simulink model "Battery_Pack_Subsystem"  (R2015a)
settings: Solver=ode45  StartTime=0.0  StopTime=300  RelTol=1e-3
libraries: fl_lib x316, nesl_utility x2
(part 1 of 2)
settings Model: Creator=satya  LastModifiedBy=satya

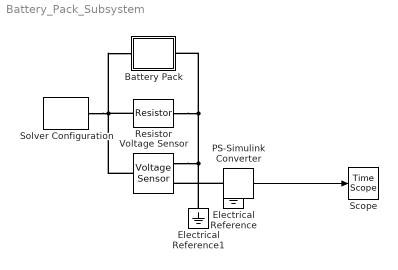
== system Battery_Pack_Subsystem ==
  Battery Pack : Subsystem
  Electrical Reference : fl_lib/Electrical/Electrical Elements/Electrical Reference
  Electrical Reference1 : fl_lib/Electrical/Electrical Elements/Electrical Reference
  PS-Simulink Converter : nesl_utility/PS-Simulink Converter  PhysicalDomain=network_engine_domain  SubClassName=ps_output  LeftPortType=input  RightPortType=output  PseudoPeriodic=off  Frequencies=[]  Unit=1  AffineConversion=off
  Resistor : fl_lib/Electrical/Electrical Elements/Resistor  R=1000 Ohm  i_specify=off  i_priority=High  i=0 A  v_specify=off  v_priority=High  v=0 V
  Scope : TimeScope
  Solver Configuration : nesl_utility/Solver Configuration  PhysicalDomain=network_engine_domain  SubClassName=solver  LeftPortType=input  RightPortType=generic  Accelerate=off  Tones=[]  Harmonics=[]  SimulateNoise=off  Profile=off  UseLocalSampling=off  EnableSwitchedLinearOptims=on  FrequencyDomain=off  UseCCode=off  RelTol=0.001  AbsTol=1e-06  MinStep=1e-09  ToWorkspace=off  RevertToSquareIcSolve=off  NumHomotopyIterations=100  DoDC=off  ResidualTolerance=1e-09  UseLocalSolver=off  LocalSolverChoice=NE_BACKWARD_EULER_ADVANCER  LocalSolverSampleTime=0.001  DoFixedCost=off  MaxNonlinIter=3  MaxModeIter=2  LinearAlgebra=Sparse  DelaysMemoryBudget=1024  AutomaticFiltering=on  FilteringTimeConstant=0.001
  Voltage Sensor : fl_lib/Electrical/Electrical Sensors/Voltage Sensor
  wires:
  PS-Simulink Converter/1 -> Scope/1
  connections:
  Voltage Sensor/RConn2 -- Battery Pack/RConn1 -- Resistor/RConn1 -- Electrical Reference1/LConn1
  Voltage Sensor/LConn1 -- Battery Pack/LConn1 -- Resistor/LConn1 -- Solver Configuration/RConn1
  PS-Simulink Converter/LConn1 -- Voltage Sensor/RConn1

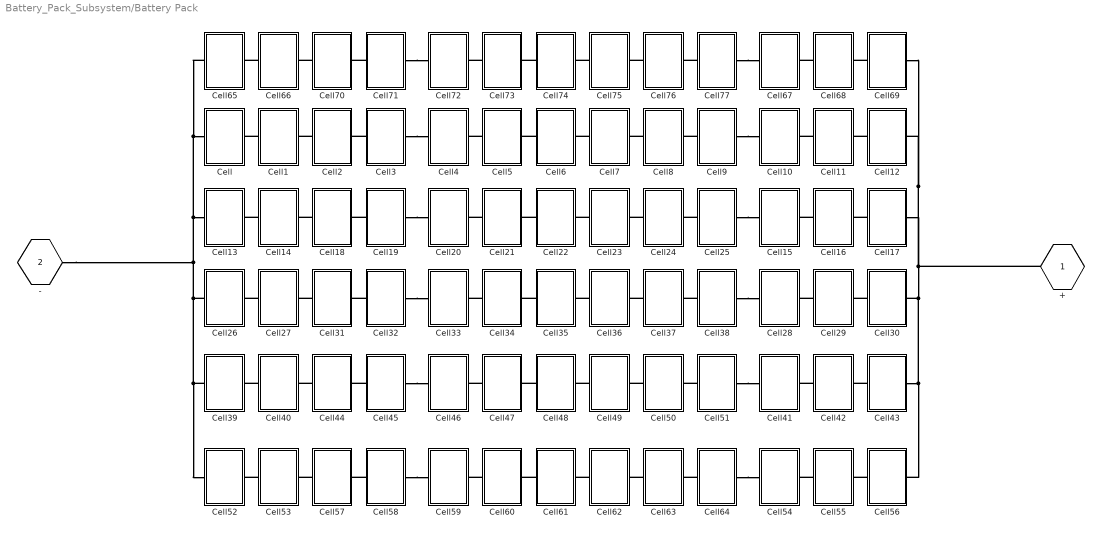
== system Battery_Pack_Subsystem/Battery Pack ==
  Cell : Subsystem
  Cell1 : Subsystem
  Cell10 : Subsystem
  Cell11 : Subsystem
  Cell12 : Subsystem
  Cell13 : Subsystem
  Cell14 : Subsystem
  Cell15 : Subsystem
  Cell16 : Subsystem
  Cell17 : Subsystem
  Cell18 : Subsystem
  Cell19 : Subsystem
  Cell2 : Subsystem
  Cell20 : Subsystem
  Cell21 : Subsystem
  Cell22 : Subsystem
  Cell23 : Subsystem
  Cell24 : Subsystem
  Cell25 : Subsystem
  Cell26 : Subsystem
  Cell27 : Subsystem
  Cell28 : Subsystem
  Cell29 : Subsystem
  Cell3 : Subsystem
  Cell30 : Subsystem
  Cell31 : Subsystem
  Cell32 : Subsystem
  Cell33 : Subsystem
  Cell34 : Subsystem
  Cell35 : Subsystem
  Cell36 : Subsystem
  Cell37 : Subsystem
  Cell38 : Subsystem
  Cell39 : Subsystem
  Cell4 : Subsystem
  Cell40 : Subsystem
  Cell41 : Subsystem
  Cell42 : Subsystem
  Cell43 : Subsystem
  Cell44 : Subsystem
  Cell45 : Subsystem
  Cell46 : Subsystem
  Cell47 : Subsystem
  Cell48 : Subsystem
  Cell49 : Subsystem
  Cell5 : Subsystem
  Cell50 : Subsystem
  Cell51 : Subsystem
  Cell52 : Subsystem
  Cell53 : Subsystem
  Cell54 : Subsystem
  Cell55 : Subsystem
  Cell56 : Subsystem
  Cell57 : Subsystem
  Cell58 : Subsystem
  Cell59 : Subsystem
  Cell6 : Subsystem
  Cell60 : Subsystem
  Cell61 : Subsystem
  Cell62 : Subsystem
  Cell63 : Subsystem
  Cell64 : Subsystem
  Cell65 : Subsystem
  Cell66 : Subsystem
  Cell67 : Subsystem
  Cell68 : Subsystem
  Cell69 : Subsystem
  Cell7 : Subsystem
  Cell70 : Subsystem
  Cell71 : Subsystem
  Cell72 : Subsystem
  Cell73 : Subsystem
  Cell74 : Subsystem
  Cell75 : Subsystem
  Cell76 : Subsystem
  Cell77 : Subsystem
  Cell8 : Subsystem
  Cell9 : Subsystem
  + : PMIOPort  Port=1  Side=Left
  - : PMIOPort  Port=2  Side=Right
  connections:
  Cell60/LConn1 -- Cell59/RConn1
  Cell62/LConn1 -- Cell61/RConn1
  Cell57/LConn1 -- Cell53/RConn1
  Cell64/RConn1 -- Cell54/LConn1
  Cell58/RConn1 -- Cell59/LConn1
  Cell64/LConn1 -- Cell63/RConn1
  Cell55/LConn1 -- Cell54/RConn1
  Cell63/LConn1 -- Cell62/RConn1
  Cell53/LConn1 -- Cell52/RConn1
  Cell58/LConn1 -- Cell57/RConn1
  Cell56/LConn1 -- Cell55/RConn1
  Cell61/LConn1 -- Cell60/RConn1
  Cell29/LConn1 -- Cell28/RConn1
  Cell31/LConn1 -- Cell27/RConn1
  Cell34/LConn1 -- Cell33/RConn1
  Cell35/LConn1 -- Cell34/RConn1
  Cell36/LConn1 -- Cell35/RConn1
  Cell32/LConn1 -- Cell31/RConn1
  Cell37/LConn1 -- Cell36/RConn1
  Cell38/RConn1 -- Cell28/LConn1
  Cell38/LConn1 -- Cell37/RConn1
  Cell51/LConn1 -- Cell50/RConn1
  Cell50/LConn1 -- Cell49/RConn1
  Cell51/RConn1 -- Cell41/LConn1
  Cell27/LConn1 -- Cell26/RConn1
  Cell40/LConn1 -- Cell39/RConn1
  Cell43/LConn1 -- Cell42/RConn1
  Cell45/RConn1 -- Cell46/LConn1
  Cell32/RConn1 -- Cell33/LConn1
  Cell30/LConn1 -- Cell29/RConn1
  Cell5/LConn1 -- Cell4/RConn1
  Cell47/LConn1 -- Cell46/RConn1
  Cell44/LConn1 -- Cell40/RConn1
  Cell48/LConn1 -- Cell47/RConn1
  Cell42/LConn1 -- Cell41/RConn1
  Cell49/LConn1 -- Cell48/RConn1
  Cell45/LConn1 -- Cell44/RConn1
  Cell2/LConn1 -- Cell1/RConn1
  Cell3/LConn1 -- Cell2/RConn1
  Cell77/LConn1 -- Cell76/RConn1
  Cell77/RConn1 -- Cell67/LConn1
  Cell71/LConn1 -- Cell70/RConn1
  Cell66/LConn1 -- Cell65/RConn1
  Cell76/LConn1 -- Cell75/RConn1
  Cell69/LConn1 -- Cell68/RConn1
  Cell71/RConn1 -- Cell72/LConn1
  Cell74/LConn1 -- Cell73/RConn1
  Cell73/LConn1 -- Cell72/RConn1
  Cell68/LConn1 -- Cell67/RConn1
  Cell70/LConn1 -- Cell66/RConn1
  Cell75/LConn1 -- Cell74/RConn1
  Cell6/LConn1 -- Cell5/RConn1
  Cell11/LConn1 -- Cell10/RConn1
  Cell7/LConn1 -- Cell6/RConn1
  Cell8/LConn1 -- Cell7/RConn1
  Cell9/RConn1 -- Cell10/LConn1
  Cell9/LConn1 -- Cell8/RConn1
  Cell43/RConn1 -- Cell56/RConn1 -- +/RConn1 -- Cell17/RConn1 -- Cell69/RConn1 -- Cell12/RConn1 -- Cell30/RConn1
  Cell3/RConn1 -- Cell4/LConn1
  Cell12/LConn1 -- Cell11/RConn1
  Cell25/RConn1 -- Cell15/LConn1
  Cell25/LConn1 -- Cell24/RConn1
  Cell16/LConn1 -- Cell15/RConn1
  Cell23/LConn1 -- Cell22/RConn1
  Cell24/LConn1 -- Cell23/RConn1
  Cell21/LConn1 -- Cell20/RConn1
  Cell17/LConn1 -- Cell16/RConn1
  Cell14/LConn1 -- Cell13/RConn1
  Cell22/LConn1 -- Cell21/RConn1
  Cell18/LConn1 -- Cell14/RConn1
  Cell19/LConn1 -- Cell18/RConn1
  Cell19/RConn1 -- Cell20/LConn1
  Cell1/LConn1 -- Cell/RConn1
  Cell39/LConn1 -- Cell52/LConn1 -- Cell26/LConn1 -- -/RConn1 -- Cell65/LConn1 -- Cell/LConn1 -- Cell13/LConn1

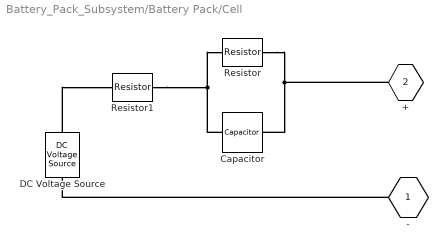
== system Battery_Pack_Subsystem/Battery Pack/Cell ==
  Capacitor : fl_lib/Electrical/Electrical Elements/Capacitor  c=5000 F  r=1e-6 Ohm  g=0 1/Ohm  i_specify=off  i_priority=High  i=0 A  v_specify=off  v_priority=High  v=0 V  vc_specify=off  vc_priority=High  vc=0 V
  DC Voltage Source : fl_lib/Electrical/Electrical Sources/DC Voltage Source  v0=4 V
  Resistor : fl_lib/Electrical/Electrical Elements/Resistor  R=0.005 Ohm  i_specify=off  i_priority=High  i=0 A  v_specify=off  v_priority=High  v=0 V
  Resistor1 : fl_lib/Electrical/Electrical Elements/Resistor  R=0.1 Ohm  i_specify=off  i_priority=High  i=0 A  v_specify=off  v_priority=High  v=0 V
  - : PMIOPort  Port=1  Side=Left
  + : PMIOPort  Port=2  Side=Right
  connections:
  Capacitor/LConn1 -- Resistor1/RConn1 -- Resistor/LConn1
  Resistor/RConn1 -- +/RConn1 -- Capacitor/RConn1
  DC Voltage Source/LConn1 -- Resistor1/LConn1
  -/RConn1 -- DC Voltage Source/RConn1

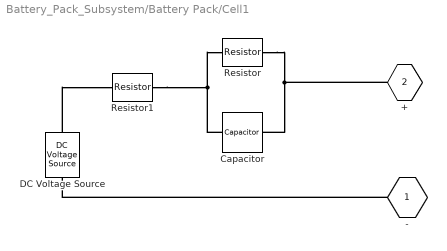
== system Battery_Pack_Subsystem/Battery Pack/Cell1 ==
  Capacitor : fl_lib/Electrical/Electrical Elements/Capacitor  c=5000 F  r=1e-6 Ohm  g=0 1/Ohm  i_specify=off  i_priority=High  i=0 A  v_specify=off  v_priority=High  v=0 V  vc_specify=off  vc_priority=High  vc=0 V
  DC Voltage Source : fl_lib/Electrical/Electrical Sources/DC Voltage Source  v0=4 V
  Resistor : fl_lib/Electrical/Electrical Elements/Resistor  R=0.005 Ohm  i_specify=off  i_priority=High  i=0 A  v_specify=off  v_priority=High  v=0 V
  Resistor1 : fl_lib/Electrical/Electrical Elements/Resistor  R=0.1 Ohm  i_specify=off  i_priority=High  i=0 A  v_specify=off  v_priority=High  v=0 V
  - : PMIOPort  Port=1  Side=Left
  + : PMIOPort  Port=2  Side=Right
  connections:
  Capacitor/LConn1 -- Resistor/LConn1 -- Resistor1/RConn1
  Resistor/RConn1 -- Capacitor/RConn1 -- +/RConn1
  DC Voltage Source/LConn1 -- Resistor1/LConn1
  -/RConn1 -- DC Voltage Source/RConn1

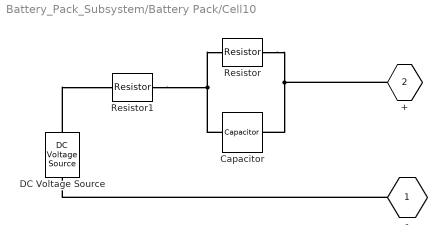
== system Battery_Pack_Subsystem/Battery Pack/Cell10 ==
  Capacitor : fl_lib/Electrical/Electrical Elements/Capacitor  c=5000 F  r=1e-6 Ohm  g=0 1/Ohm  i_specify=off  i_priority=High  i=0 A  v_specify=off  v_priority=High  v=0 V  vc_specify=off  vc_priority=High  vc=0 V
  DC Voltage Source : fl_lib/Electrical/Electrical Sources/DC Voltage Source  v0=4 V
  Resistor : fl_lib/Electrical/Electrical Elements/Resistor  R=0.005 Ohm  i_specify=off  i_priority=High  i=0 A  v_specify=off  v_priority=High  v=0 V
  Resistor1 : fl_lib/Electrical/Electrical Elements/Resistor  R=0.1 Ohm  i_specify=off  i_priority=High  i=0 A  v_specify=off  v_priority=High  v=0 V
  - : PMIOPort  Port=1  Side=Left
  + : PMIOPort  Port=2  Side=Right
  connections:
  Capacitor/LConn1 -- Resistor/LConn1 -- Resistor1/RConn1
  Resistor/RConn1 -- Capacitor/RConn1 -- +/RConn1
  DC Voltage Source/LConn1 -- Resistor1/LConn1
  -/RConn1 -- DC Voltage Source/RConn1

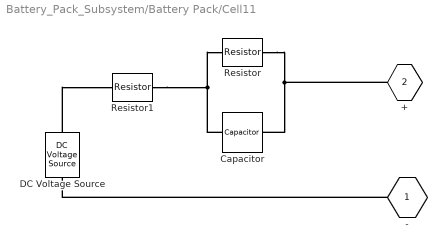
== system Battery_Pack_Subsystem/Battery Pack/Cell11 ==
  Capacitor : fl_lib/Electrical/Electrical Elements/Capacitor  c=5000 F  r=1e-6 Ohm  g=0 1/Ohm  i_specify=off  i_priority=High  i=0 A  v_specify=off  v_priority=High  v=0 V  vc_specify=off  vc_priority=High  vc=0 V
  DC Voltage Source : fl_lib/Electrical/Electrical Sources/DC Voltage Source  v0=4 V
  Resistor : fl_lib/Electrical/Electrical Elements/Resistor  R=0.005 Ohm  i_specify=off  i_priority=High  i=0 A  v_specify=off  v_priority=High  v=0 V
  Resistor1 : fl_lib/Electrical/Electrical Elements/Resistor  R=0.1 Ohm  i_specify=off  i_priority=High  i=0 A  v_specify=off  v_priority=High  v=0 V
  - : PMIOPort  Port=1  Side=Left
  + : PMIOPort  Port=2  Side=Right
  connections:
  Capacitor/LConn1 -- Resistor/LConn1 -- Resistor1/RConn1
  Resistor/RConn1 -- Capacitor/RConn1 -- +/RConn1
  DC Voltage Source/LConn1 -- Resistor1/LConn1
  -/RConn1 -- DC Voltage Source/RConn1

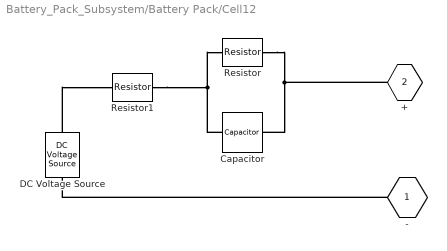
== system Battery_Pack_Subsystem/Battery Pack/Cell12 ==
  Capacitor : fl_lib/Electrical/Electrical Elements/Capacitor  c=5000 F  r=1e-6 Ohm  g=0 1/Ohm  i_specify=off  i_priority=High  i=0 A  v_specify=off  v_priority=High  v=0 V  vc_specify=off  vc_priority=High  vc=0 V
  DC Voltage Source : fl_lib/Electrical/Electrical Sources/DC Voltage Source  v0=4 V
  Resistor : fl_lib/Electrical/Electrical Elements/Resistor  R=0.005 Ohm  i_specify=off  i_priority=High  i=0 A  v_specify=off  v_priority=High  v=0 V
  Resistor1 : fl_lib/Electrical/Electrical Elements/Resistor  R=0.1 Ohm  i_specify=off  i_priority=High  i=0 A  v_specify=off  v_priority=High  v=0 V
  - : PMIOPort  Port=1  Side=Left
  + : PMIOPort  Port=2  Side=Right
  connections:
  Capacitor/LConn1 -- Resistor/LConn1 -- Resistor1/RConn1
  Resistor/RConn1 -- Capacitor/RConn1 -- +/RConn1
  DC Voltage Source/LConn1 -- Resistor1/LConn1
  -/RConn1 -- DC Voltage Source/RConn1

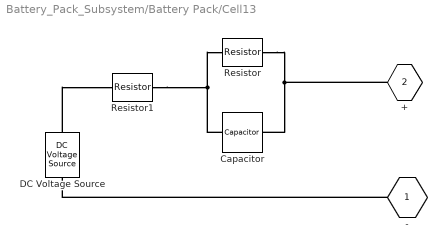
== system Battery_Pack_Subsystem/Battery Pack/Cell13 ==
  Capacitor : fl_lib/Electrical/Electrical Elements/Capacitor  c=5000 F  r=1e-6 Ohm  g=0 1/Ohm  i_specify=off  i_priority=High  i=0 A  v_specify=off  v_priority=High  v=0 V  vc_specify=off  vc_priority=High  vc=0 V
  DC Voltage Source : fl_lib/Electrical/Electrical Sources/DC Voltage Source  v0=4 V
  Resistor : fl_lib/Electrical/Electrical Elements/Resistor  R=0.005 Ohm  i_specify=off  i_priority=High  i=0 A  v_specify=off  v_priority=High  v=0 V
  Resistor1 : fl_lib/Electrical/Electrical Elements/Resistor  R=0.1 Ohm  i_specify=off  i_priority=High  i=0 A  v_specify=off  v_priority=High  v=0 V
  - : PMIOPort  Port=1  Side=Left
  + : PMIOPort  Port=2  Side=Right
  connections:
  Capacitor/LConn1 -- Resistor/LConn1 -- Resistor1/RConn1
  Resistor/RConn1 -- Capacitor/RConn1 -- +/RConn1
  DC Voltage Source/LConn1 -- Resistor1/LConn1
  -/RConn1 -- DC Voltage Source/RConn1

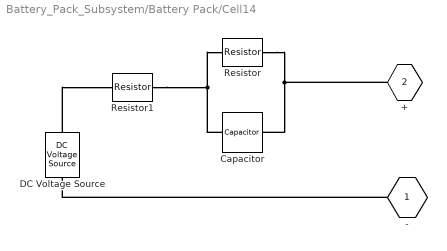
== system Battery_Pack_Subsystem/Battery Pack/Cell14 ==
  Capacitor : fl_lib/Electrical/Electrical Elements/Capacitor  c=5000 F  r=1e-6 Ohm  g=0 1/Ohm  i_specify=off  i_priority=High  i=0 A  v_specify=off  v_priority=High  v=0 V  vc_specify=off  vc_priority=High  vc=0 V
  DC Voltage Source : fl_lib/Electrical/Electrical Sources/DC Voltage Source  v0=4 V
  Resistor : fl_lib/Electrical/Electrical Elements/Resistor  R=0.005 Ohm  i_specify=off  i_priority=High  i=0 A  v_specify=off  v_priority=High  v=0 V
  Resistor1 : fl_lib/Electrical/Electrical Elements/Resistor  R=0.1 Ohm  i_specify=off  i_priority=High  i=0 A  v_specify=off  v_priority=High  v=0 V
  - : PMIOPort  Port=1  Side=Left
  + : PMIOPort  Port=2  Side=Right
  connections:
  Capacitor/LConn1 -- Resistor/LConn1 -- Resistor1/RConn1
  Resistor/RConn1 -- Capacitor/RConn1 -- +/RConn1
  DC Voltage Source/LConn1 -- Resistor1/LConn1
  -/RConn1 -- DC Voltage Source/RConn1

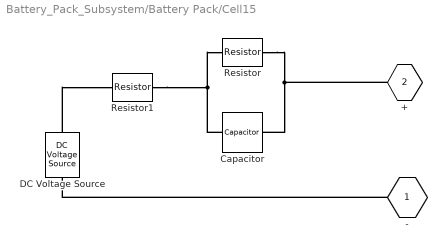
== system Battery_Pack_Subsystem/Battery Pack/Cell15 ==
  Capacitor : fl_lib/Electrical/Electrical Elements/Capacitor  c=5000 F  r=1e-6 Ohm  g=0 1/Ohm  i_specify=off  i_priority=High  i=0 A  v_specify=off  v_priority=High  v=0 V  vc_specify=off  vc_priority=High  vc=0 V
  DC Voltage Source : fl_lib/Electrical/Electrical Sources/DC Voltage Source  v0=4 V
  Resistor : fl_lib/Electrical/Electrical Elements/Resistor  R=0.005 Ohm  i_specify=off  i_priority=High  i=0 A  v_specify=off  v_priority=High  v=0 V
  Resistor1 : fl_lib/Electrical/Electrical Elements/Resistor  R=0.1 Ohm  i_specify=off  i_priority=High  i=0 A  v_specify=off  v_priority=High  v=0 V
  - : PMIOPort  Port=1  Side=Left
  + : PMIOPort  Port=2  Side=Right
  connections:
  Capacitor/LConn1 -- Resistor/LConn1 -- Resistor1/RConn1
  Resistor/RConn1 -- Capacitor/RConn1 -- +/RConn1
  DC Voltage Source/LConn1 -- Resistor1/LConn1
  -/RConn1 -- DC Voltage Source/RConn1

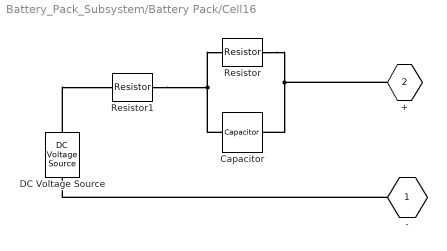
== system Battery_Pack_Subsystem/Battery Pack/Cell16 ==
  Capacitor : fl_lib/Electrical/Electrical Elements/Capacitor  c=5000 F  r=1e-6 Ohm  g=0 1/Ohm  i_specify=off  i_priority=High  i=0 A  v_specify=off  v_priority=High  v=0 V  vc_specify=off  vc_priority=High  vc=0 V
  DC Voltage Source : fl_lib/Electrical/Electrical Sources/DC Voltage Source  v0=4 V
  Resistor : fl_lib/Electrical/Electrical Elements/Resistor  R=0.005 Ohm  i_specify=off  i_priority=High  i=0 A  v_specify=off  v_priority=High  v=0 V
  Resistor1 : fl_lib/Electrical/Electrical Elements/Resistor  R=0.1 Ohm  i_specify=off  i_priority=High  i=0 A  v_specify=off  v_priority=High  v=0 V
  - : PMIOPort  Port=1  Side=Left
  + : PMIOPort  Port=2  Side=Right
  connections:
  Capacitor/LConn1 -- Resistor/LConn1 -- Resistor1/RConn1
  Resistor/RConn1 -- Capacitor/RConn1 -- +/RConn1
  DC Voltage Source/LConn1 -- Resistor1/LConn1
  -/RConn1 -- DC Voltage Source/RConn1

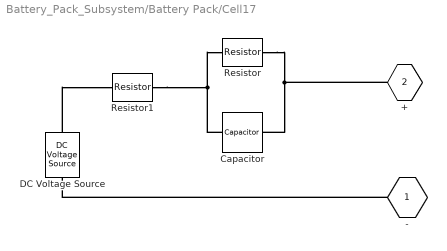
== system Battery_Pack_Subsystem/Battery Pack/Cell17 ==
  Capacitor : fl_lib/Electrical/Electrical Elements/Capacitor  c=5000 F  r=1e-6 Ohm  g=0 1/Ohm  i_specify=off  i_priority=High  i=0 A  v_specify=off  v_priority=High  v=0 V  vc_specify=off  vc_priority=High  vc=0 V
  DC Voltage Source : fl_lib/Electrical/Electrical Sources/DC Voltage Source  v0=4 V
  Resistor : fl_lib/Electrical/Electrical Elements/Resistor  R=0.005 Ohm  i_specify=off  i_priority=High  i=0 A  v_specify=off  v_priority=High  v=0 V
  Resistor1 : fl_lib/Electrical/Electrical Elements/Resistor  R=0.1 Ohm  i_specify=off  i_priority=High  i=0 A  v_specify=off  v_priority=High  v=0 V
  - : PMIOPort  Port=1  Side=Left
  + : PMIOPort  Port=2  Side=Right
  connections:
  Capacitor/LConn1 -- Resistor/LConn1 -- Resistor1/RConn1
  Resistor/RConn1 -- Capacitor/RConn1 -- +/RConn1
  DC Voltage Source/LConn1 -- Resistor1/LConn1
  -/RConn1 -- DC Voltage Source/RConn1

== system Battery_Pack_Subsystem/Battery Pack/Cell18 ==
  Capacitor : fl_lib/Electrical/Electrical Elements/Capacitor  c=5000 F  r=1e-6 Ohm  g=0 1/Ohm  i_specify=off  i_priority=High  i=0 A  v_specify=off  v_priority=High  v=0 V  vc_specify=off  vc_priority=High  vc=0 V
  DC Voltage Source : fl_lib/Electrical/Electrical Sources/DC Voltage Source  v0=4 V
  Resistor : fl_lib/Electrical/Electrical Elements/Resistor  R=0.005 Ohm  i_specify=off  i_priority=High  i=0 A  v_specify=off  v_priority=High  v=0 V
  Resistor1 : fl_lib/Electrical/Electrical Elements/Resistor  R=0.1 Ohm  i_specify=off  i_priority=High  i=0 A  v_specify=off  v_priority=High  v=0 V
  - : PMIOPort  Port=1  Side=Left
  + : PMIOPort  Port=2  Side=Right
  connections:
  Capacitor/LConn1 -- Resistor/LConn1 -- Resistor1/RConn1
  Resistor/RConn1 -- Capacitor/RConn1 -- +/RConn1
  DC Voltage Source/LConn1 -- Resistor1/LConn1
  -/RConn1 -- DC Voltage Source/RConn1

== system Battery_Pack_Subsystem/Battery Pack/Cell19 ==
  Capacitor : fl_lib/Electrical/Electrical Elements/Capacitor  c=5000 F  r=1e-6 Ohm  g=0 1/Ohm  i_specify=off  i_priority=High  i=0 A  v_specify=off  v_priority=High  v=0 V  vc_specify=off  vc_priority=High  vc=0 V
  DC Voltage Source : fl_lib/Electrical/Electrical Sources/DC Voltage Source  v0=4 V
  Resistor : fl_lib/Electrical/Electrical Elements/Resistor  R=0.005 Ohm  i_specify=off  i_priority=High  i=0 A  v_specify=off  v_priority=High  v=0 V
  Resistor1 : fl_lib/Electrical/Electrical Elements/Resistor  R=0.1 Ohm  i_specify=off  i_priority=High  i=0 A  v_specify=off  v_priority=High  v=0 V
  - : PMIOPort  Port=1  Side=Left
  + : PMIOPort  Port=2  Side=Right
  connections:
  Capacitor/LConn1 -- Resistor/LConn1 -- Resistor1/RConn1
  Resistor/RConn1 -- Capacitor/RConn1 -- +/RConn1
  DC Voltage Source/LConn1 -- Resistor1/LConn1
  -/RConn1 -- DC Voltage Source/RConn1

== system Battery_Pack_Subsystem/Battery Pack/Cell2 ==
  Capacitor : fl_lib/Electrical/Electrical Elements/Capacitor  c=5000 F  r=1e-6 Ohm  g=0 1/Ohm  i_specify=off  i_priority=High  i=0 A  v_specify=off  v_priority=High  v=0 V  vc_specify=off  vc_priority=High  vc=0 V
  DC Voltage Source : fl_lib/Electrical/Electrical Sources/DC Voltage Source  v0=4 V
  Resistor : fl_lib/Electrical/Electrical Elements/Resistor  R=0.005 Ohm  i_specify=off  i_priority=High  i=0 A  v_specify=off  v_priority=High  v=0 V
  Resistor1 : fl_lib/Electrical/Electrical Elements/Resistor  R=0.1 Ohm  i_specify=off  i_priority=High  i=0 A  v_specify=off  v_priority=High  v=0 V
  - : PMIOPort  Port=1  Side=Left
  + : PMIOPort  Port=2  Side=Right
  connections:
  Capacitor/LConn1 -- Resistor/LConn1 -- Resistor1/RConn1
  Resistor/RConn1 -- Capacitor/RConn1 -- +/RConn1
  DC Voltage Source/LConn1 -- Resistor1/LConn1
  -/RConn1 -- DC Voltage Source/RConn1

== system Battery_Pack_Subsystem/Battery Pack/Cell20 ==
  Capacitor : fl_lib/Electrical/Electrical Elements/Capacitor  c=5000 F  r=1e-6 Ohm  g=0 1/Ohm  i_specify=off  i_priority=High  i=0 A  v_specify=off  v_priority=High  v=0 V  vc_specify=off  vc_priority=High  vc=0 V
  DC Voltage Source : fl_lib/Electrical/Electrical Sources/DC Voltage Source  v0=4 V
  Resistor : fl_lib/Electrical/Electrical Elements/Resistor  R=0.005 Ohm  i_specify=off  i_priority=High  i=0 A  v_specify=off  v_priority=High  v=0 V
  Resistor1 : fl_lib/Electrical/Electrical Elements/Resistor  R=0.1 Ohm  i_specify=off  i_priority=High  i=0 A  v_specify=off  v_priority=High  v=0 V
  - : PMIOPort  Port=1  Side=Left
  + : PMIOPort  Port=2  Side=Right
  connections:
  Capacitor/LConn1 -- Resistor/LConn1 -- Resistor1/RConn1
  Resistor/RConn1 -- Capacitor/RConn1 -- +/RConn1
  DC Voltage Source/LConn1 -- Resistor1/LConn1
  -/RConn1 -- DC Voltage Source/RConn1

== system Battery_Pack_Subsystem/Battery Pack/Cell21 ==
  Capacitor : fl_lib/Electrical/Electrical Elements/Capacitor  c=5000 F  r=1e-6 Ohm  g=0 1/Ohm  i_specify=off  i_priority=High  i=0 A  v_specify=off  v_priority=High  v=0 V  vc_specify=off  vc_priority=High  vc=0 V
  DC Voltage Source : fl_lib/Electrical/Electrical Sources/DC Voltage Source  v0=4 V
  Resistor : fl_lib/Electrical/Electrical Elements/Resistor  R=0.005 Ohm  i_specify=off  i_priority=High  i=0 A  v_specify=off  v_priority=High  v=0 V
  Resistor1 : fl_lib/Electrical/Electrical Elements/Resistor  R=0.1 Ohm  i_specify=off  i_priority=High  i=0 A  v_specify=off  v_priority=High  v=0 V
  - : PMIOPort  Port=1  Side=Left
  + : PMIOPort  Port=2  Side=Right
  connections:
  Capacitor/LConn1 -- Resistor/LConn1 -- Resistor1/RConn1
  Resistor/RConn1 -- Capacitor/RConn1 -- +/RConn1
  DC Voltage Source/LConn1 -- Resistor1/LConn1
  -/RConn1 -- DC Voltage Source/RConn1

== system Battery_Pack_Subsystem/Battery Pack/Cell22 ==
  Capacitor : fl_lib/Electrical/Electrical Elements/Capacitor  c=5000 F  r=1e-6 Ohm  g=0 1/Ohm  i_specify=off  i_priority=High  i=0 A  v_specify=off  v_priority=High  v=0 V  vc_specify=off  vc_priority=High  vc=0 V
  DC Voltage Source : fl_lib/Electrical/Electrical Sources/DC Voltage Source  v0=4 V
  Resistor : fl_lib/Electrical/Electrical Elements/Resistor  R=0.005 Ohm  i_specify=off  i_priority=High  i=0 A  v_specify=off  v_priority=High  v=0 V
  Resistor1 : fl_lib/Electrical/Electrical Elements/Resistor  R=0.1 Ohm  i_specify=off  i_priority=High  i=0 A  v_specify=off  v_priority=High  v=0 V
  - : PMIOPort  Port=1  Side=Left
  + : PMIOPort  Port=2  Side=Right
  connections:
  Capacitor/LConn1 -- Resistor/LConn1 -- Resistor1/RConn1
  Resistor/RConn1 -- Capacitor/RConn1 -- +/RConn1
  DC Voltage Source/LConn1 -- Resistor1/LConn1
  -/RConn1 -- DC Voltage Source/RConn1

== system Battery_Pack_Subsystem/Battery Pack/Cell23 ==
  Capacitor : fl_lib/Electrical/Electrical Elements/Capacitor  c=5000 F  r=1e-6 Ohm  g=0 1/Ohm  i_specify=off  i_priority=High  i=0 A  v_specify=off  v_priority=High  v=0 V  vc_specify=off  vc_priority=High  vc=0 V
  DC Voltage Source : fl_lib/Electrical/Electrical Sources/DC Voltage Source  v0=4 V
  Resistor : fl_lib/Electrical/Electrical Elements/Resistor  R=0.005 Ohm  i_specify=off  i_priority=High  i=0 A  v_specify=off  v_priority=High  v=0 V
  Resistor1 : fl_lib/Electrical/Electrical Elements/Resistor  R=0.1 Ohm  i_specify=off  i_priority=High  i=0 A  v_specify=off  v_priority=High  v=0 V
  - : PMIOPort  Port=1  Side=Left
  + : PMIOPort  Port=2  Side=Right
  connections:
  Capacitor/LConn1 -- Resistor/LConn1 -- Resistor1/RConn1
  Resistor/RConn1 -- Capacitor/RConn1 -- +/RConn1
  DC Voltage Source/LConn1 -- Resistor1/LConn1
  -/RConn1 -- DC Voltage Source/RConn1

== system Battery_Pack_Subsystem/Battery Pack/Cell24 ==
  Capacitor : fl_lib/Electrical/Electrical Elements/Capacitor  c=5000 F  r=1e-6 Ohm  g=0 1/Ohm  i_specify=off  i_priority=High  i=0 A  v_specify=off  v_priority=High  v=0 V  vc_specify=off  vc_priority=High  vc=0 V
  DC Voltage Source : fl_lib/Electrical/Electrical Sources/DC Voltage Source  v0=4 V
  Resistor : fl_lib/Electrical/Electrical Elements/Resistor  R=0.005 Ohm  i_specify=off  i_priority=High  i=0 A  v_specify=off  v_priority=High  v=0 V
  Resistor1 : fl_lib/Electrical/Electrical Elements/Resistor  R=0.1 Ohm  i_specify=off  i_priority=High  i=0 A  v_specify=off  v_priority=High  v=0 V
  - : PMIOPort  Port=1  Side=Left
  + : PMIOPort  Port=2  Side=Right
  connections:
  Capacitor/LConn1 -- Resistor/LConn1 -- Resistor1/RConn1
  Resistor/RConn1 -- Capacitor/RConn1 -- +/RConn1
  DC Voltage Source/LConn1 -- Resistor1/LConn1
  -/RConn1 -- DC Voltage Source/RConn1

== system Battery_Pack_Subsystem/Battery Pack/Cell25 ==
  Capacitor : fl_lib/Electrical/Electrical Elements/Capacitor  c=5000 F  r=1e-6 Ohm  g=0 1/Ohm  i_specify=off  i_priority=High  i=0 A  v_specify=off  v_priority=High  v=0 V  vc_specify=off  vc_priority=High  vc=0 V
  DC Voltage Source : fl_lib/Electrical/Electrical Sources/DC Voltage Source  v0=4 V
  Resistor : fl_lib/Electrical/Electrical Elements/Resistor  R=0.005 Ohm  i_specify=off  i_priority=High  i=0 A  v_specify=off  v_priority=High  v=0 V
  Resistor1 : fl_lib/Electrical/Electrical Elements/Resistor  R=0.1 Ohm  i_specify=off  i_priority=High  i=0 A  v_specify=off  v_priority=High  v=0 V
  - : PMIOPort  Port=1  Side=Left
  + : PMIOPort  Port=2  Side=Right
  connections:
  Capacitor/LConn1 -- Resistor/LConn1 -- Resistor1/RConn1
  Resistor/RConn1 -- Capacitor/RConn1 -- +/RConn1
  DC Voltage Source/LConn1 -- Resistor1/LConn1
  -/RConn1 -- DC Voltage Source/RConn1

== system Battery_Pack_Subsystem/Battery Pack/Cell26 ==
  Capacitor : fl_lib/Electrical/Electrical Elements/Capacitor  c=5000 F  r=1e-6 Ohm  g=0 1/Ohm  i_specify=off  i_priority=High  i=0 A  v_specify=off  v_priority=High  v=0 V  vc_specify=off  vc_priority=High  vc=0 V
  DC Voltage Source : fl_lib/Electrical/Electrical Sources/DC Voltage Source  v0=4 V
  Resistor : fl_lib/Electrical/Electrical Elements/Resistor  R=0.005 Ohm  i_specify=off  i_priority=High  i=0 A  v_specify=off  v_priority=High  v=0 V
  Resistor1 : fl_lib/Electrical/Electrical Elements/Resistor  R=0.1 Ohm  i_specify=off  i_priority=High  i=0 A  v_specify=off  v_priority=High  v=0 V
  - : PMIOPort  Port=1  Side=Left
  + : PMIOPort  Port=2  Side=Right
  connections:
  Capacitor/LConn1 -- Resistor/LConn1 -- Resistor1/RConn1
  Resistor/RConn1 -- Capacitor/RConn1 -- +/RConn1
  DC Voltage Source/LConn1 -- Resistor1/LConn1
  -/RConn1 -- DC Voltage Source/RConn1

== system Battery_Pack_Subsystem/Battery Pack/Cell27 ==
  Capacitor : fl_lib/Electrical/Electrical Elements/Capacitor  c=5000 F  r=1e-6 Ohm  g=0 1/Ohm  i_specify=off  i_priority=High  i=0 A  v_specify=off  v_priority=High  v=0 V  vc_specify=off  vc_priority=High  vc=0 V
  DC Voltage Source : fl_lib/Electrical/Electrical Sources/DC Voltage Source  v0=4 V
  Resistor : fl_lib/Electrical/Electrical Elements/Resistor  R=0.005 Ohm  i_specify=off  i_priority=High  i=0 A  v_specify=off  v_priority=High  v=0 V
  Resistor1 : fl_lib/Electrical/Electrical Elements/Resistor  R=0.1 Ohm  i_specify=off  i_priority=High  i=0 A  v_specify=off  v_priority=High  v=0 V
  - : PMIOPort  Port=1  Side=Left
  + : PMIOPort  Port=2  Side=Right
  connections:
  Capacitor/LConn1 -- Resistor/LConn1 -- Resistor1/RConn1
  Resistor/RConn1 -- Capacitor/RConn1 -- +/RConn1
  DC Voltage Source/LConn1 -- Resistor1/LConn1
  -/RConn1 -- DC Voltage Source/RConn1

== system Battery_Pack_Subsystem/Battery Pack/Cell28 ==
  Capacitor : fl_lib/Electrical/Electrical Elements/Capacitor  c=5000 F  r=1e-6 Ohm  g=0 1/Ohm  i_specify=off  i_priority=High  i=0 A  v_specify=off  v_priority=High  v=0 V  vc_specify=off  vc_priority=High  vc=0 V
  DC Voltage Source : fl_lib/Electrical/Electrical Sources/DC Voltage Source  v0=4 V
  Resistor : fl_lib/Electrical/Electrical Elements/Resistor  R=0.005 Ohm  i_specify=off  i_priority=High  i=0 A  v_specify=off  v_priority=High  v=0 V
  Resistor1 : fl_lib/Electrical/Electrical Elements/Resistor  R=0.1 Ohm  i_specify=off  i_priority=High  i=0 A  v_specify=off  v_priority=High  v=0 V
  - : PMIOPort  Port=1  Side=Left
  + : PMIOPort  Port=2  Side=Right
  connections:
  Capacitor/LConn1 -- Resistor/LConn1 -- Resistor1/RConn1
  Resistor/RConn1 -- Capacitor/RConn1 -- +/RConn1
  DC Voltage Source/LConn1 -- Resistor1/LConn1
  -/RConn1 -- DC Voltage Source/RConn1

== system Battery_Pack_Subsystem/Battery Pack/Cell29 ==
  Capacitor : fl_lib/Electrical/Electrical Elements/Capacitor  c=5000 F  r=1e-6 Ohm  g=0 1/Ohm  i_specify=off  i_priority=High  i=0 A  v_specify=off  v_priority=High  v=0 V  vc_specify=off  vc_priority=High  vc=0 V
  DC Voltage Source : fl_lib/Electrical/Electrical Sources/DC Voltage Source  v0=4 V
  Resistor : fl_lib/Electrical/Electrical Elements/Resistor  R=0.005 Ohm  i_specify=off  i_priority=High  i=0 A  v_specify=off  v_priority=High  v=0 V
  Resistor1 : fl_lib/Electrical/Electrical Elements/Resistor  R=0.1 Ohm  i_specify=off  i_priority=High  i=0 A  v_specify=off  v_priority=High  v=0 V
  - : PMIOPort  Port=1  Side=Left
  + : PMIOPort  Port=2  Side=Right
  connections:
  Capacitor/LConn1 -- Resistor/LConn1 -- Resistor1/RConn1
  Resistor/RConn1 -- Capacitor/RConn1 -- +/RConn1
  DC Voltage Source/LConn1 -- Resistor1/LConn1
  -/RConn1 -- DC Voltage Source/RConn1

== system Battery_Pack_Subsystem/Battery Pack/Cell3 ==
  Capacitor : fl_lib/Electrical/Electrical Elements/Capacitor  c=5000 F  r=1e-6 Ohm  g=0 1/Ohm  i_specify=off  i_priority=High  i=0 A  v_specify=off  v_priority=High  v=0 V  vc_specify=off  vc_priority=High  vc=0 V
  DC Voltage Source : fl_lib/Electrical/Electrical Sources/DC Voltage Source  v0=4 V
  Resistor : fl_lib/Electrical/Electrical Elements/Resistor  R=0.005 Ohm  i_specify=off  i_priority=High  i=0 A  v_specify=off  v_priority=High  v=0 V
  Resistor1 : fl_lib/Electrical/Electrical Elements/Resistor  R=0.1 Ohm  i_specify=off  i_priority=High  i=0 A  v_specify=off  v_priority=High  v=0 V
  - : PMIOPort  Port=1  Side=Left
  + : PMIOPort  Port=2  Side=Right
  connections:
  Capacitor/LConn1 -- Resistor/LConn1 -- Resistor1/RConn1
  Resistor/RConn1 -- Capacitor/RConn1 -- +/RConn1
  DC Voltage Source/LConn1 -- Resistor1/LConn1
  -/RConn1 -- DC Voltage Source/RConn1

== system Battery_Pack_Subsystem/Battery Pack/Cell30 ==
  Capacitor : fl_lib/Electrical/Electrical Elements/Capacitor  c=5000 F  r=1e-6 Ohm  g=0 1/Ohm  i_specify=off  i_priority=High  i=0 A  v_specify=off  v_priority=High  v=0 V  vc_specify=off  vc_priority=High  vc=0 V
  DC Voltage Source : fl_lib/Electrical/Electrical Sources/DC Voltage Source  v0=4 V
  Resistor : fl_lib/Electrical/Electrical Elements/Resistor  R=0.005 Ohm  i_specify=off  i_priority=High  i=0 A  v_specify=off  v_priority=High  v=0 V
  Resistor1 : fl_lib/Electrical/Electrical Elements/Resistor  R=0.1 Ohm  i_specify=off  i_priority=High  i=0 A  v_specify=off  v_priority=High  v=0 V
  - : PMIOPort  Port=1  Side=Left
  + : PMIOPort  Port=2  Side=Right
  connections:
  Capacitor/LConn1 -- Resistor/LConn1 -- Resistor1/RConn1
  Resistor/RConn1 -- Capacitor/RConn1 -- +/RConn1
  DC Voltage Source/LConn1 -- Resistor1/LConn1
  -/RConn1 -- DC Voltage Source/RConn1

== system Battery_Pack_Subsystem/Battery Pack/Cell31 ==
  Capacitor : fl_lib/Electrical/Electrical Elements/Capacitor  c=5000 F  r=1e-6 Ohm  g=0 1/Ohm  i_specify=off  i_priority=High  i=0 A  v_specify=off  v_priority=High  v=0 V  vc_specify=off  vc_priority=High  vc=0 V
  DC Voltage Source : fl_lib/Electrical/Electrical Sources/DC Voltage Source  v0=4 V
  Resistor : fl_lib/Electrical/Electrical Elements/Resistor  R=0.005 Ohm  i_specify=off  i_priority=High  i=0 A  v_specify=off  v_priority=High  v=0 V
  Resistor1 : fl_lib/Electrical/Electrical Elements/Resistor  R=0.1 Ohm  i_specify=off  i_priority=High  i=0 A  v_specify=off  v_priority=High  v=0 V
  - : PMIOPort  Port=1  Side=Left
  + : PMIOPort  Port=2  Side=Right
  connections:
  Capacitor/LConn1 -- Resistor/LConn1 -- Resistor1/RConn1
  Resistor/RConn1 -- Capacitor/RConn1 -- +/RConn1
  DC Voltage Source/LConn1 -- Resistor1/LConn1
  -/RConn1 -- DC Voltage Source/RConn1

== system Battery_Pack_Subsystem/Battery Pack/Cell32 ==
  Capacitor : fl_lib/Electrical/Electrical Elements/Capacitor  c=5000 F  r=1e-6 Ohm  g=0 1/Ohm  i_specify=off  i_priority=High  i=0 A  v_specify=off  v_priority=High  v=0 V  vc_specify=off  vc_priority=High  vc=0 V
  DC Voltage Source : fl_lib/Electrical/Electrical Sources/DC Voltage Source  v0=4 V
  Resistor : fl_lib/Electrical/Electrical Elements/Resistor  R=0.005 Ohm  i_specify=off  i_priority=High  i=0 A  v_specify=off  v_priority=High  v=0 V
  Resistor1 : fl_lib/Electrical/Electrical Elements/Resistor  R=0.1 Ohm  i_specify=off  i_priority=High  i=0 A  v_specify=off  v_priority=High  v=0 V
  - : PMIOPort  Port=1  Side=Left
  + : PMIOPort  Port=2  Side=Right
  connections:
  Capacitor/LConn1 -- Resistor/LConn1 -- Resistor1/RConn1
  Resistor/RConn1 -- Capacitor/RConn1 -- +/RConn1
  DC Voltage Source/LConn1 -- Resistor1/LConn1
  -/RConn1 -- DC Voltage Source/RConn1

== system Battery_Pack_Subsystem/Battery Pack/Cell33 ==
  Capacitor : fl_lib/Electrical/Electrical Elements/Capacitor  c=5000 F  r=1e-6 Ohm  g=0 1/Ohm  i_specify=off  i_priority=High  i=0 A  v_specify=off  v_priority=High  v=0 V  vc_specify=off  vc_priority=High  vc=0 V
  DC Voltage Source : fl_lib/Electrical/Electrical Sources/DC Voltage Source  v0=4 V
  Resistor : fl_lib/Electrical/Electrical Elements/Resistor  R=0.005 Ohm  i_specify=off  i_priority=High  i=0 A  v_specify=off  v_priority=High  v=0 V
  Resistor1 : fl_lib/Electrical/Electrical Elements/Resistor  R=0.1 Ohm  i_specify=off  i_priority=High  i=0 A  v_specify=off  v_priority=High  v=0 V
  - : PMIOPort  Port=1  Side=Left
  + : PMIOPort  Port=2  Side=Right
  connections:
  Capacitor/LConn1 -- Resistor/LConn1 -- Resistor1/RConn1
  Resistor/RConn1 -- Capacitor/RConn1 -- +/RConn1
  DC Voltage Source/LConn1 -- Resistor1/LConn1
  -/RConn1 -- DC Voltage Source/RConn1

== system Battery_Pack_Subsystem/Battery Pack/Cell34 ==
  Capacitor : fl_lib/Electrical/Electrical Elements/Capacitor  c=5000 F  r=1e-6 Ohm  g=0 1/Ohm  i_specify=off  i_priority=High  i=0 A  v_specify=off  v_priority=High  v=0 V  vc_specify=off  vc_priority=High  vc=0 V
  DC Voltage Source : fl_lib/Electrical/Electrical Sources/DC Voltage Source  v0=4 V
  Resistor : fl_lib/Electrical/Electrical Elements/Resistor  R=0.005 Ohm  i_specify=off  i_priority=High  i=0 A  v_specify=off  v_priority=High  v=0 V
  Resistor1 : fl_lib/Electrical/Electrical Elements/Resistor  R=0.1 Ohm  i_specify=off  i_priority=High  i=0 A  v_specify=off  v_priority=High  v=0 V
  - : PMIOPort  Port=1  Side=Left
  + : PMIOPort  Port=2  Side=Right
  connections:
  Capacitor/LConn1 -- Resistor/LConn1 -- Resistor1/RConn1
  Resistor/RConn1 -- Capacitor/RConn1 -- +/RConn1
  DC Voltage Source/LConn1 -- Resistor1/LConn1
  -/RConn1 -- DC Voltage Source/RConn1

== system Battery_Pack_Subsystem/Battery Pack/Cell35 ==
  Capacitor : fl_lib/Electrical/Electrical Elements/Capacitor  c=5000 F  r=1e-6 Ohm  g=0 1/Ohm  i_specify=off  i_priority=High  i=0 A  v_specify=off  v_priority=High  v=0 V  vc_specify=off  vc_priority=High  vc=0 V
  DC Voltage Source : fl_lib/Electrical/Electrical Sources/DC Voltage Source  v0=4 V
  Resistor : fl_lib/Electrical/Electrical Elements/Resistor  R=0.005 Ohm  i_specify=off  i_priority=High  i=0 A  v_specify=off  v_priority=High  v=0 V
  Resistor1 : fl_lib/Electrical/Electrical Elements/Resistor  R=0.1 Ohm  i_specify=off  i_priority=High  i=0 A  v_specify=off  v_priority=High  v=0 V
  - : PMIOPort  Port=1  Side=Left
  + : PMIOPort  Port=2  Side=Right
  connections:
  Capacitor/LConn1 -- Resistor/LConn1 -- Resistor1/RConn1
  Resistor/RConn1 -- Capacitor/RConn1 -- +/RConn1
  DC Voltage Source/LConn1 -- Resistor1/LConn1
  -/RConn1 -- DC Voltage Source/RConn1

== system Battery_Pack_Subsystem/Battery Pack/Cell36 ==
  Capacitor : fl_lib/Electrical/Electrical Elements/Capacitor  c=5000 F  r=1e-6 Ohm  g=0 1/Ohm  i_specify=off  i_priority=High  i=0 A  v_specify=off  v_priority=High  v=0 V  vc_specify=off  vc_priority=High  vc=0 V
  DC Voltage Source : fl_lib/Electrical/Electrical Sources/DC Voltage Source  v0=4 V
  Resistor : fl_lib/Electrical/Electrical Elements/Resistor  R=0.005 Ohm  i_specify=off  i_priority=High  i=0 A  v_specify=off  v_priority=High  v=0 V
  Resistor1 : fl_lib/Electrical/Electrical Elements/Resistor  R=0.1 Ohm  i_specify=off  i_priority=High  i=0 A  v_specify=off  v_priority=High  v=0 V
  - : PMIOPort  Port=1  Side=Left
  + : PMIOPort  Port=2  Side=Right
  connections:
  Capacitor/LConn1 -- Resistor/LConn1 -- Resistor1/RConn1
  Resistor/RConn1 -- Capacitor/RConn1 -- +/RConn1
  DC Voltage Source/LConn1 -- Resistor1/LConn1
  -/RConn1 -- DC Voltage Source/RConn1

== system Battery_Pack_Subsystem/Battery Pack/Cell37 ==
  Capacitor : fl_lib/Electrical/Electrical Elements/Capacitor  c=5000 F  r=1e-6 Ohm  g=0 1/Ohm  i_specify=off  i_priority=High  i=0 A  v_specify=off  v_priority=High  v=0 V  vc_specify=off  vc_priority=High  vc=0 V
  DC Voltage Source : fl_lib/Electrical/Electrical Sources/DC Voltage Source  v0=4 V
  Resistor : fl_lib/Electrical/Electrical Elements/Resistor  R=0.005 Ohm  i_specify=off  i_priority=High  i=0 A  v_specify=off  v_priority=High  v=0 V
  Resistor1 : fl_lib/Electrical/Electrical Elements/Resistor  R=0.1 Ohm  i_specify=off  i_priority=High  i=0 A  v_specify=off  v_priority=High  v=0 V
  - : PMIOPort  Port=1  Side=Left
  + : PMIOPort  Port=2  Side=Right
  connections:
  Capacitor/LConn1 -- Resistor/LConn1 -- Resistor1/RConn1
  Resistor/RConn1 -- Capacitor/RConn1 -- +/RConn1
  DC Voltage Source/LConn1 -- Resistor1/LConn1
  -/RConn1 -- DC Voltage Source/RConn1

== system Battery_Pack_Subsystem/Battery Pack/Cell38 ==
  Capacitor : fl_lib/Electrical/Electrical Elements/Capacitor  c=5000 F  r=1e-6 Ohm  g=0 1/Ohm  i_specify=off  i_priority=High  i=0 A  v_specify=off  v_priority=High  v=0 V  vc_specify=off  vc_priority=High  vc=0 V
  DC Voltage Source : fl_lib/Electrical/Electrical Sources/DC Voltage Source  v0=4 V
  Resistor : fl_lib/Electrical/Electrical Elements/Resistor  R=0.005 Ohm  i_specify=off  i_priority=High  i=0 A  v_specify=off  v_priority=High  v=0 V
  Resistor1 : fl_lib/Electrical/Electrical Elements/Resistor  R=0.1 Ohm  i_specify=off  i_priority=High  i=0 A  v_specify=off  v_priority=High  v=0 V
  - : PMIOPort  Port=1  Side=Left
  + : PMIOPort  Port=2  Side=Right
  connections:
  Capacitor/LConn1 -- Resistor/LConn1 -- Resistor1/RConn1
  Resistor/RConn1 -- Capacitor/RConn1 -- +/RConn1
  DC Voltage Source/LConn1 -- Resistor1/LConn1
  -/RConn1 -- DC Voltage Source/RConn1

== system Battery_Pack_Subsystem/Battery Pack/Cell39 ==
  Capacitor : fl_lib/Electrical/Electrical Elements/Capacitor  c=5000 F  r=1e-6 Ohm  g=0 1/Ohm  i_specify=off  i_priority=High  i=0 A  v_specify=off  v_priority=High  v=0 V  vc_specify=off  vc_priority=High  vc=0 V
  DC Voltage Source : fl_lib/Electrical/Electrical Sources/DC Voltage Source  v0=4 V
  Resistor : fl_lib/Electrical/Electrical Elements/Resistor  R=0.005 Ohm  i_specify=off  i_priority=High  i=0 A  v_specify=off  v_priority=High  v=0 V
  Resistor1 : fl_lib/Electrical/Electrical Elements/Resistor  R=0.1 Ohm  i_specify=off  i_priority=High  i=0 A  v_specify=off  v_priority=High  v=0 V
  - : PMIOPort  Port=1  Side=Left
  + : PMIOPort  Port=2  Side=Right
  connections:
  Capacitor/LConn1 -- Resistor/LConn1 -- Resistor1/RConn1
  Resistor/RConn1 -- Capacitor/RConn1 -- +/RConn1
  DC Voltage Source/LConn1 -- Resistor1/LConn1
  -/RConn1 -- DC Voltage Source/RConn1

== system Battery_Pack_Subsystem/Battery Pack/Cell4 ==
  Capacitor : fl_lib/Electrical/Electrical Elements/Capacitor  c=5000 F  r=1e-6 Ohm  g=0 1/Ohm  i_specify=off  i_priority=High  i=0 A  v_specify=off  v_priority=High  v=0 V  vc_specify=off  vc_priority=High  vc=0 V
  DC Voltage Source : fl_lib/Electrical/Electrical Sources/DC Voltage Source  v0=4 V
  Resistor : fl_lib/Electrical/Electrical Elements/Resistor  R=0.005 Ohm  i_specify=off  i_priority=High  i=0 A  v_specify=off  v_priority=High  v=0 V
  Resistor1 : fl_lib/Electrical/Electrical Elements/Resistor  R=0.1 Ohm  i_specify=off  i_priority=High  i=0 A  v_specify=off  v_priority=High  v=0 V
  - : PMIOPort  Port=1  Side=Left
  + : PMIOPort  Port=2  Side=Right
  connections:
  Capacitor/LConn1 -- Resistor/LConn1 -- Resistor1/RConn1
  Resistor/RConn1 -- Capacitor/RConn1 -- +/RConn1
  DC Voltage Source/LConn1 -- Resistor1/LConn1
  -/RConn1 -- DC Voltage Source/RConn1

== system Battery_Pack_Subsystem/Battery Pack/Cell40 ==
  Capacitor : fl_lib/Electrical/Electrical Elements/Capacitor  c=5000 F  r=1e-6 Ohm  g=0 1/Ohm  i_specify=off  i_priority=High  i=0 A  v_specify=off  v_priority=High  v=0 V  vc_specify=off  vc_priority=High  vc=0 V
  DC Voltage Source : fl_lib/Electrical/Electrical Sources/DC Voltage Source  v0=4 V
  Resistor : fl_lib/Electrical/Electrical Elements/Resistor  R=0.005 Ohm  i_specify=off  i_priority=High  i=0 A  v_specify=off  v_priority=High  v=0 V
  Resistor1 : fl_lib/Electrical/Electrical Elements/Resistor  R=0.1 Ohm  i_specify=off  i_priority=High  i=0 A  v_specify=off  v_priority=High  v=0 V
  - : PMIOPort  Port=1  Side=Left
  + : PMIOPort  Port=2  Side=Right
  connections:
  Capacitor/LConn1 -- Resistor/LConn1 -- Resistor1/RConn1
  Resistor/RConn1 -- Capacitor/RConn1 -- +/RConn1
  DC Voltage Source/LConn1 -- Resistor1/LConn1
  -/RConn1 -- DC Voltage Source/RConn1

== system Battery_Pack_Subsystem/Battery Pack/Cell41 ==
  Capacitor : fl_lib/Electrical/Electrical Elements/Capacitor  c=5000 F  r=1e-6 Ohm  g=0 1/Ohm  i_specify=off  i_priority=High  i=0 A  v_specify=off  v_priority=High  v=0 V  vc_specify=off  vc_priority=High  vc=0 V
  DC Voltage Source : fl_lib/Electrical/Electrical Sources/DC Voltage Source  v0=4 V
  Resistor : fl_lib/Electrical/Electrical Elements/Resistor  R=0.005 Ohm  i_specify=off  i_priority=High  i=0 A  v_specify=off  v_priority=High  v=0 V
  Resistor1 : fl_lib/Electrical/Electrical Elements/Resistor  R=0.1 Ohm  i_specify=off  i_priority=High  i=0 A  v_specify=off  v_priority=High  v=0 V
  - : PMIOPort  Port=1  Side=Left
  + : PMIOPort  Port=2  Side=Right
  connections:
  Capacitor/LConn1 -- Resistor/LConn1 -- Resistor1/RConn1
  Resistor/RConn1 -- Capacitor/RConn1 -- +/RConn1
  DC Voltage Source/LConn1 -- Resistor1/LConn1
  -/RConn1 -- DC Voltage Source/RConn1

== system Battery_Pack_Subsystem/Battery Pack/Cell42 ==
  Capacitor : fl_lib/Electrical/Electrical Elements/Capacitor  c=5000 F  r=1e-6 Ohm  g=0 1/Ohm  i_specify=off  i_priority=High  i=0 A  v_specify=off  v_priority=High  v=0 V  vc_specify=off  vc_priority=High  vc=0 V
  DC Voltage Source : fl_lib/Electrical/Electrical Sources/DC Voltage Source  v0=4 V
  Resistor : fl_lib/Electrical/Electrical Elements/Resistor  R=0.005 Ohm  i_specify=off  i_priority=High  i=0 A  v_specify=off  v_priority=High  v=0 V
  Resistor1 : fl_lib/Electrical/Electrical Elements/Resistor  R=0.1 Ohm  i_specify=off  i_priority=High  i=0 A  v_specify=off  v_priority=High  v=0 V
  - : PMIOPort  Port=1  Side=Left
  + : PMIOPort  Port=2  Side=Right
  connections:
  Capacitor/LConn1 -- Resistor/LConn1 -- Resistor1/RConn1
  Resistor/RConn1 -- Capacitor/RConn1 -- +/RConn1
  DC Voltage Source/LConn1 -- Resistor1/LConn1
  -/RConn1 -- DC Voltage Source/RConn1

== system Battery_Pack_Subsystem/Battery Pack/Cell43 ==
  Capacitor : fl_lib/Electrical/Electrical Elements/Capacitor  c=5000 F  r=1e-6 Ohm  g=0 1/Ohm  i_specify=off  i_priority=High  i=0 A  v_specify=off  v_priority=High  v=0 V  vc_specify=off  vc_priority=High  vc=0 V
  DC Voltage Source : fl_lib/Electrical/Electrical Sources/DC Voltage Source  v0=4 V
  Resistor : fl_lib/Electrical/Electrical Elements/Resistor  R=0.005 Ohm  i_specify=off  i_priority=High  i=0 A  v_specify=off  v_priority=High  v=0 V
  Resistor1 : fl_lib/Electrical/Electrical Elements/Resistor  R=0.1 Ohm  i_specify=off  i_priority=High  i=0 A  v_specify=off  v_priority=High  v=0 V
  - : PMIOPort  Port=1  Side=Left
  + : PMIOPort  Port=2  Side=Right
  connections:
  Capacitor/LConn1 -- Resistor/LConn1 -- Resistor1/RConn1
  Resistor/RConn1 -- Capacitor/RConn1 -- +/RConn1
  DC Voltage Source/LConn1 -- Resistor1/LConn1
  -/RConn1 -- DC Voltage Source/RConn1

== system Battery_Pack_Subsystem/Battery Pack/Cell44 ==
  Capacitor : fl_lib/Electrical/Electrical Elements/Capacitor  c=5000 F  r=1e-6 Ohm  g=0 1/Ohm  i_specify=off  i_priority=High  i=0 A  v_specify=off  v_priority=High  v=0 V  vc_specify=off  vc_priority=High  vc=0 V
  DC Voltage Source : fl_lib/Electrical/Electrical Sources/DC Voltage Source  v0=4 V
  Resistor : fl_lib/Electrical/Electrical Elements/Resistor  R=0.005 Ohm  i_specify=off  i_priority=High  i=0 A  v_specify=off  v_priority=High  v=0 V
  Resistor1 : fl_lib/Electrical/Electrical Elements/Resistor  R=0.1 Ohm  i_specify=off  i_priority=High  i=0 A  v_specify=off  v_priority=High  v=0 V
  - : PMIOPort  Port=1  Side=Left
  + : PMIOPort  Port=2  Side=Right
  connections:
  Capacitor/LConn1 -- Resistor/LConn1 -- Resistor1/RConn1
  Resistor/RConn1 -- Capacitor/RConn1 -- +/RConn1
  DC Voltage Source/LConn1 -- Resistor1/LConn1
  -/RConn1 -- DC Voltage Source/RConn1

== system Battery_Pack_Subsystem/Battery Pack/Cell45 ==
  Capacitor : fl_lib/Electrical/Electrical Elements/Capacitor  c=5000 F  r=1e-6 Ohm  g=0 1/Ohm  i_specify=off  i_priority=High  i=0 A  v_specify=off  v_priority=High  v=0 V  vc_specify=off  vc_priority=High  vc=0 V
  DC Voltage Source : fl_lib/Electrical/Electrical Sources/DC Voltage Source  v0=4 V
  Resistor : fl_lib/Electrical/Electrical Elements/Resistor  R=0.005 Ohm  i_specify=off  i_priority=High  i=0 A  v_specify=off  v_priority=High  v=0 V
  Resistor1 : fl_lib/Electrical/Electrical Elements/Resistor  R=0.1 Ohm  i_specify=off  i_priority=High  i=0 A  v_specify=off  v_priority=High  v=0 V
  - : PMIOPort  Port=1  Side=Left
  + : PMIOPort  Port=2  Side=Right
  connections:
  Capacitor/LConn1 -- Resistor/LConn1 -- Resistor1/RConn1
  Resistor/RConn1 -- Capacitor/RConn1 -- +/RConn1
  DC Voltage Source/LConn1 -- Resistor1/LConn1
  -/RConn1 -- DC Voltage Source/RConn1

== system Battery_Pack_Subsystem/Battery Pack/Cell46 ==
  Capacitor : fl_lib/Electrical/Electrical Elements/Capacitor  c=5000 F  r=1e-6 Ohm  g=0 1/Ohm  i_specify=off  i_priority=High  i=0 A  v_specify=off  v_priority=High  v=0 V  vc_specify=off  vc_priority=High  vc=0 V
  DC Voltage Source : fl_lib/Electrical/Electrical Sources/DC Voltage Source  v0=4 V
  Resistor : fl_lib/Electrical/Electrical Elements/Resistor  R=0.005 Ohm  i_specify=off  i_priority=High  i=0 A  v_specify=off  v_priority=High  v=0 V
  Resistor1 : fl_lib/Electrical/Electrical Elements/Resistor  R=0.1 Ohm  i_specify=off  i_priority=High  i=0 A  v_specify=off  v_priority=High  v=0 V
  - : PMIOPort  Port=1  Side=Left
  + : PMIOPort  Port=2  Side=Right
  connections:
  Capacitor/LConn1 -- Resistor/LConn1 -- Resistor1/RConn1
  Resistor/RConn1 -- Capacitor/RConn1 -- +/RConn1
  DC Voltage Source/LConn1 -- Resistor1/LConn1
  -/RConn1 -- DC Voltage Source/RConn1

== system Battery_Pack_Subsystem/Battery Pack/Cell47 ==
  Capacitor : fl_lib/Electrical/Electrical Elements/Capacitor  c=5000 F  r=1e-6 Ohm  g=0 1/Ohm  i_specify=off  i_priority=High  i=0 A  v_specify=off  v_priority=High  v=0 V  vc_specify=off  vc_priority=High  vc=0 V
  DC Voltage Source : fl_lib/Electrical/Electrical Sources/DC Voltage Source  v0=4 V
  Resistor : fl_lib/Electrical/Electrical Elements/Resistor  R=0.005 Ohm  i_specify=off  i_priority=High  i=0 A  v_specify=off  v_priority=High  v=0 V
  Resistor1 : fl_lib/Electrical/Electrical Elements/Resistor  R=0.1 Ohm  i_specify=off  i_priority=High  i=0 A  v_specify=off  v_priority=High  v=0 V
  - : PMIOPort  Port=1  Side=Left
  + : PMIOPort  Port=2  Side=Right
  connections:
  Capacitor/LConn1 -- Resistor/LConn1 -- Resistor1/RConn1
  Resistor/RConn1 -- Capacitor/RConn1 -- +/RConn1
  DC Voltage Source/LConn1 -- Resistor1/LConn1
  -/RConn1 -- DC Voltage Source/RConn1

== system Battery_Pack_Subsystem/Battery Pack/Cell48 ==
  Capacitor : fl_lib/Electrical/Electrical Elements/Capacitor  c=5000 F  r=1e-6 Ohm  g=0 1/Ohm  i_specify=off  i_priority=High  i=0 A  v_specify=off  v_priority=High  v=0 V  vc_specify=off  vc_priority=High  vc=0 V
  DC Voltage Source : fl_lib/Electrical/Electrical Sources/DC Voltage Source  v0=4 V
  Resistor : fl_lib/Electrical/Electrical Elements/Resistor  R=0.005 Ohm  i_specify=off  i_priority=High  i=0 A  v_specify=off  v_priority=High  v=0 V
  Resistor1 : fl_lib/Electrical/Electrical Elements/Resistor  R=0.1 Ohm  i_specify=off  i_priority=High  i=0 A  v_specify=off  v_priority=High  v=0 V
  - : PMIOPort  Port=1  Side=Left
  + : PMIOPort  Port=2  Side=Right
  connections:
  Capacitor/LConn1 -- Resistor/LConn1 -- Resistor1/RConn1
  Resistor/RConn1 -- Capacitor/RConn1 -- +/RConn1
  DC Voltage Source/LConn1 -- Resistor1/LConn1
  -/RConn1 -- DC Voltage Source/RConn1

== system Battery_Pack_Subsystem/Battery Pack/Cell49 ==
  Capacitor : fl_lib/Electrical/Electrical Elements/Capacitor  c=5000 F  r=1e-6 Ohm  g=0 1/Ohm  i_specify=off  i_priority=High  i=0 A  v_specify=off  v_priority=High  v=0 V  vc_specify=off  vc_priority=High  vc=0 V
  DC Voltage Source : fl_lib/Electrical/Electrical Sources/DC Voltage Source  v0=4 V
  Resistor : fl_lib/Electrical/Electrical Elements/Resistor  R=0.005 Ohm  i_specify=off  i_priority=High  i=0 A  v_specify=off  v_priority=High  v=0 V
  Resistor1 : fl_lib/Electrical/Electrical Elements/Resistor  R=0.1 Ohm  i_specify=off  i_priority=High  i=0 A  v_specify=off  v_priority=High  v=0 V
  - : PMIOPort  Port=1  Side=Left
  + : PMIOPort  Port=2  Side=Right
  connections:
  Capacitor/LConn1 -- Resistor/LConn1 -- Resistor1/RConn1
  Resistor/RConn1 -- Capacitor/RConn1 -- +/RConn1
  DC Voltage Source/LConn1 -- Resistor1/LConn1
  -/RConn1 -- DC Voltage Source/RConn1

== system Battery_Pack_Subsystem/Battery Pack/Cell5 ==
  Capacitor : fl_lib/Electrical/Electrical Elements/Capacitor  c=5000 F  r=1e-6 Ohm  g=0 1/Ohm  i_specify=off  i_priority=High  i=0 A  v_specify=off  v_priority=High  v=0 V  vc_specify=off  vc_priority=High  vc=0 V
  DC Voltage Source : fl_lib/Electrical/Electrical Sources/DC Voltage Source  v0=4 V
  Resistor : fl_lib/Electrical/Electrical Elements/Resistor  R=0.005 Ohm  i_specify=off  i_priority=High  i=0 A  v_specify=off  v_priority=High  v=0 V
  Resistor1 : fl_lib/Electrical/Electrical Elements/Resistor  R=0.1 Ohm  i_specify=off  i_priority=High  i=0 A  v_specify=off  v_priority=High  v=0 V
  - : PMIOPort  Port=1  Side=Left
  + : PMIOPort  Port=2  Side=Right
  connections:
  Capacitor/LConn1 -- Resistor/LConn1 -- Resistor1/RConn1
  Resistor/RConn1 -- Capacitor/RConn1 -- +/RConn1
  DC Voltage Source/LConn1 -- Resistor1/LConn1
  -/RConn1 -- DC Voltage Source/RConn1
